simulink model "gm_sampleModel1448_3_sub"  (R2023a)
settings: Solver=VariableStepAuto  StartTime=0.0  StopTime=10.0  RelTol=1e-3
libraries: simulink x1
settings Model: Creator=user1  LastModifiedBy=user1
settings OptimizationCC: BlockReduction=off  ConditionallyExecuteInputs=off
settings DebuggingCC: InheritedTsInSrcMsg=none

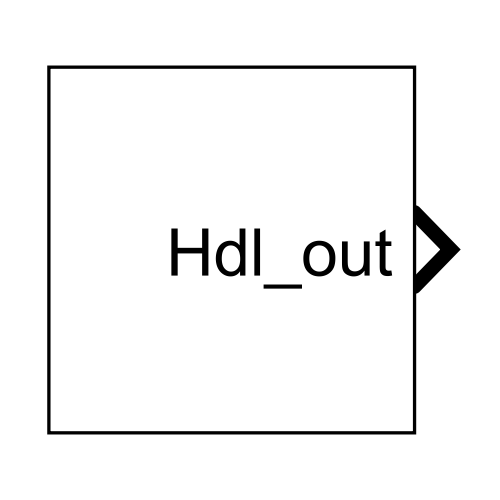
[thumbnail: Simulink's stored preview of the top-level diagram]
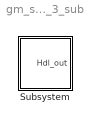
== system gm_sampleModel1448_3_sub ==
  Subsystem : Subsystem

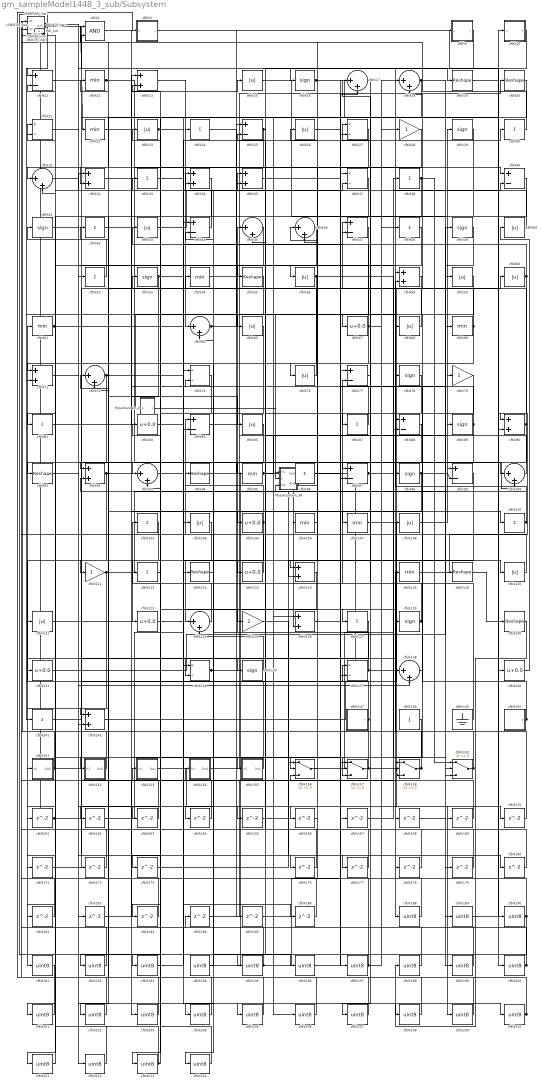
== system gm_sampleModel1448_3_sub/Subsystem ==
  Mysubsystem_3 : Subsystem
  Mysubsystem_38 : Subsystem
  cfblk10 : Subsystem  mask(Detect Rise Positive){vinit=double(0), InputProcessing=Elements as channels (sample based), OutDataTypeStr=uint8}
      mask prompts: vinit "Simulink:masks:InitialCondition_MP"; InputProcessing "Simulink:masks:InputProcessing_MP"; OutDataTypeStr "Simulink:masks:OutputDataType_MP"
      mask help: Simulink:masks:DetectRisePositive_MD
      mask init:
      | InputProcessing = 'Elements as channels (sample based)';
      | OutDataTypeStr = 'uint8';
      | vinit = double(0);
      mask TypeOptions InputProcessing: Simulink:masks:ColumnsAsChannelsFrameBased | Simulink:masks:ElementsAsChannelsSampleBased
      mask TypeOptions OutDataTypeStr: Simulink:masks:uint8 | Simulink:masks:boolean
      mask Display: fprintf('U > 0\n&  NOT\nU/z > 0')
  cfblk{17..18,31,45..46,64,72,93,100,124,138} (11 alike) : Sum  Inputs=|++  OutDataTypeStr=uint8
  cfblk101_inst : Subsystem
  cfblk102_inst : Subsystem
  cfblk{24,30,33,38,42,48,52,81,87,96,103,110,113,127,141} (15 alike) : Sum  Inputs=+  OutDataTypeStr=uint8
  cfblk{15,23,26,43,50,56,59..60,65,68,76,85,104,108,120..121} (16 alike) : Abs  OutDataTypeStr=uint8  SaturateOnIntegerOverflow=off
  cfblk{67,83,105,115,123,131,140} (7 alike) : Bias  Bias=0.0  SaturateOnIntegerOverflow=off
  cfblk{12,22,54,61,69,95,106..107,118} (9 alike) : MinMax  OutDataTypeStr=uint8
  cfblk{11,25,40,44,47,77,84,88,97,99} (10 alike) : Sum  Inputs=+-  OutDataTypeStr=uint8
  cfblk{28,79,112,125} (4 alike) : Gain  OutDataTypeStr=uint8
  cfblk{19..20,55,91,94,114,119,130} (8 alike) : Reshape
  cfblk{13,32,34..35,58,71,90,92,116,126,142} (11 alike) : Sum  OutDataTypeStr=uint8
  cfblk117_inst : Subsystem
  cfblk122_inst : Subsystem
  cfblk{16,29,41,49,53,78,89,98,128,135} (10 alike) : Signum
  cfblk129_inst : Subsystem
  cfblk{21,27,37,74,134,137} (6 alike) : Product  Inputs=*/  OutDataTypeStr=uint8  RndMeth=Zero  SaturateOnIntegerOverflow=on
  cfblk136_inst : Subsystem
  cfblk139_inst : Subsystem
  cfblk147 : Subsystem  mask(Counter Free-Running){NumBits=double(16), tsamp=double(-1)}
      mask prompts: NumBits "Simulink:masks:NumberOfBits_MP"; tsamp "Simulink:masks:SampleTime_MP"
      mask help: Simulink:masks:CounterFreeRunning_MD
  cfblk148 : Constant  OutDataTypeStr=uint8  SampleTime=-1
  cfblk149 : Ground
  cfblk14_inst : Subsystem
  cfblk150 : Subsystem  mask(Counter Free-Running){NumBits=double(16), tsamp=double(-1)}
      mask prompts: NumBits "Simulink:masks:NumberOfBits_MP"; tsamp "Simulink:masks:SampleTime_MP"
      mask help: Simulink:masks:CounterFreeRunning_MD
  cfblk151 : Subsystem
  cfblk152 : Subsystem
  cfblk153 : Subsystem
  cfblk154 : Subsystem
  cfblk155 : Subsystem
  cfblk{156..159} (4 alike) : Switch  OutDataTypeStr=uint8  SaturateOnIntegerOverflow=off  InputSameDT=off
  cfblk{161..173,176..186} (24 alike) : Delay  SampleTime=1
  cfblk{188..214} (27 alike) : DataTypeConversion  OutDataTypeStr=uint8  SaturateOnIntegerOverflow=off  RndMeth=Floor
  cfblk2 : Logic  AllPortsSameDT=off  OutDataTypeStr=boolean
  cfblk3 : Subsystem  mask(Compare To Zero){relop=<=, OutDataTypeStr=uint8, ZeroCross=on}
      mask prompts: relop "Simulink:masks:Operator_MP"; OutDataTypeStr "Simulink:masks:OutputDataType_MP"; ZeroCross "Simulink:masks:EnableZerocrossingDetection_MP"
      mask help: Simulink:masks:CompareToZero_MD
      mask init:
      | OutDataTypeStr = 'uint8';
      | ZeroCross = 'on';
      | blkName = 'sampleModel1448_3_sub/Subsystem/cfblk3';
      | relop = '<=';
      | setValue = 'fixdt(0, 8)';
      mask TypeOptions relop: == | ~= | < | <= | >= | >
      mask TypeOptions OutDataTypeStr: Simulink:masks:uint8 | Simulink:masks:boolean
      mask Callback ZeroCross: sl('zeroCrossEnable', gcbh);
      mask Display: disp([relop,' 0'])
  cfblk36_inst : Subsystem
  cfblk6 : Constant  Value=0  OutDataTypeStr=uint8  SampleTime=1
  cfblk63_inst : Subsystem
  cfblk66_inst : Subsystem
  cfblk70_inst : Subsystem
  cfblk75_inst : Subsystem
  cfblk8 : Constant  Value=0  OutDataTypeStr=uint8  SampleTime=1
  cfblk82_inst : Subsystem
  cfblk9 : Subsystem  mask(Compare To Constant){relop=<=, const=double(3), OutDataTypeStr=uint8, ZeroCross=on}
      mask prompts: relop "Simulink:masks:Operator_MP"; const "Simulink:masks:ConstantValue_MP"; OutDataTypeStr "Simulink:masks:OutputDataType_MP"; ZeroCross "Simulink:masks:EnableZerocrossingDetection_MP"
      mask help: Simulink:masks:CompareToConstant_MD
      mask init:
      | OutDataTypeStr = 'uint8';
      | ZeroCross = 'on';
      | blkName = 'sampleModel1448_3_sub/Subsystem/cfblk9';
      | const = double(3);
      | const_str = '3.0';
      | const_val = double(3);
      | relop = '<=';
      | setValue = 'fixdt(0, 8)';
      | str = '<= 3';
      mask TypeOptions relop: == | ~= | < | <= | >= | >
      mask TypeOptions OutDataTypeStr: Simulink:masks:uint8 | Simulink:masks:boolean
      mask Callback ZeroCross: sl('zeroCrossEnable', gcbh);
      mask Display: disp(str)
  Hdl_out : Outport  OutDataTypeStr=uint8  SampleTime=1
  wires:
  Mysubsystem_3/1(Out1) -> Mysubsystem_38/2(u)
  Mysubsystem_38/1(Out1) -> cfblk194/1, cfblk126/2, cfblk106/1
  Mysubsystem_38/2(Out2) -> cfblk66_inst/1(in1)
  cfblk10/1(Y) -> cfblk188/1
  cfblk100/1 -> cfblk45/2
  cfblk101_inst/1(out1) -> cfblk193/1
  cfblk102_inst/1(out1) -> cfblk168/1, cfblk22/1
  cfblk103/1 -> cfblk123/1
  cfblk104/1 -> cfblk191/1
  cfblk105/1 -> cfblk84/1, cfblk124/1
  cfblk106/1 -> cfblk46/1
  cfblk107/1 -> cfblk209/1
  cfblk108/1 -> cfblk29/1
  cfblk11/1 -> cfblk126/1
  cfblk110/1 -> cfblk58/2, Mysubsystem_38/3(In3)
  cfblk112/1 -> cfblk99/1, cfblk151/1(In1)
  cfblk113/1 -> cfblk213/1
  cfblk114/1 -> cfblk134/2
  cfblk115/1 -> cfblk94/1
  cfblk116/1 -> cfblk173/1
  cfblk117_inst/1(out1) -> cfblk69/1
  cfblk118/1 -> cfblk90/1
  cfblk119/1 -> cfblk130/1
  cfblk12/1 -> cfblk67/1, cfblk100/2
  cfblk120/1 -> cfblk129_inst/1(in1)
  cfblk121/1 -> cfblk156/2
  cfblk122_inst/1(out1) -> cfblk197/1
  cfblk123/1 -> cfblk127/1
  cfblk124/1 -> cfblk103/1
  cfblk125/1 -> cfblk177/1
  cfblk126/1 -> cfblk167/1
  cfblk127/1 -> cfblk201/1
  cfblk128/1 -> cfblk77/2, cfblk27/1
  cfblk129_inst/1(out1) -> cfblk114/1
  cfblk13/1 -> cfblk64/1
  cfblk130/1 -> cfblk198/1
  cfblk131/1 -> cfblk59/1
  cfblk134/1 -> cfblk20/1, cfblk54/1
  cfblk135/1 -> cfblk124/2
  cfblk136_inst/1(out1) -> cfblk203/1
  cfblk137/1 -> cfblk45/1, cfblk34/1
  cfblk138/1 -> cfblk96/1
  cfblk139_inst/1(out1) -> cfblk200/1
  cfblk14_inst/1(out1) -> cfblk19/1, cfblk11/1
  cfblk140/1 -> cfblk50/1
  cfblk141/1 -> cfblk60/1
  cfblk142/1 -> cfblk49/1
  cfblk147/1(y) -> cfblk44/2, cfblk211/1
  cfblk148/1 -> cfblk157/3
  cfblk149/1 -> cfblk53/1
  cfblk15/1 -> cfblk189/1
  cfblk150/1(y) -> cfblk92/2, cfblk78/1
  cfblk151/1(Out1) -> cfblk75_inst/2(in2), cfblk176/1
  cfblk152/1(Out1) -> cfblk75_inst/1(in1)
  cfblk153/1(Out1) -> cfblk166/1
  cfblk154/1(Out1) -> cfblk88/1
  cfblk155/1(Out1) -> cfblk61/1
  cfblk156/1 -> cfblk38/1
  cfblk157/1 -> cfblk158/3, cfblk155/1(In1)
  cfblk158/1 -> cfblk70_inst/1(in1), cfblk31/2
  cfblk159/1 -> cfblk2/1, cfblk118/1
  cfblk16/1 -> cfblk27/2, cfblk179/1
  cfblk161/1 -> cfblk156/1, Hdl_out/1
  cfblk162/1 -> cfblk37/2
  cfblk163/1 -> cfblk72/1
  cfblk164/1 -> cfblk63_inst/2(in2)
  cfblk165/1 -> cfblk77/1
  cfblk166/1 -> cfblk46/2
  cfblk167/1 -> cfblk40/2
  cfblk168/1 -> cfblk199/1
  cfblk169/1 -> cfblk13/2
  cfblk17/1 -> cfblk87/1
  cfblk170/1 -> cfblk34/2
  cfblk171/1 -> cfblk137/1
  cfblk172/1 -> cfblk117_inst/2(in2)
  cfblk173/1 -> cfblk158/2
  cfblk176/1 -> cfblk64/2
  cfblk177/1 -> cfblk25/2
  cfblk178/1 -> cfblk70_inst/2(in2)
  cfblk179/1 -> cfblk93/2
  cfblk18/1 -> cfblk97/1, cfblk32/2, cfblk100/1, cfblk183/1, cfblk24/1
  cfblk180/1 -> cfblk134/1
  cfblk181/1 -> cfblk129_inst/2(in2)
  cfblk182/1 -> cfblk156/3
  cfblk183/1 -> cfblk36_inst/2(in2)
  cfblk184/1 -> cfblk17/2
  cfblk185/1 -> cfblk157/1
  cfblk186/1 -> cfblk2/2
  cfblk188/1 -> cfblk26/1
  cfblk189/1 -> cfblk10/1(U)
  cfblk19/1 -> cfblk140/1
  cfblk190/1 -> cfblk83/1, cfblk214/1
  cfblk191/1 -> cfblk3/1(u)
  cfblk192/1 -> cfblk66_inst/2(in2)
  cfblk193/1 -> cfblk74/1
  cfblk194/1 -> cfblk74/2
  cfblk195/1 -> cfblk97/2, cfblk36_inst/1(in1)
  cfblk196/1 -> cfblk79/1
  cfblk197/1 -> cfblk82_inst/1(in1), cfblk18/1, cfblk37/1
  cfblk198/1 -> cfblk122_inst/1(in1)
  cfblk199/1 -> cfblk122_inst/2(in2)
  cfblk2/1 -> cfblk157/2
  cfblk20/1 -> cfblk95/1
  cfblk200/1 -> cfblk117_inst/1(in1), cfblk184/1, cfblk154/1(In1)
  cfblk201/1 -> cfblk139_inst/1(in1)
  cfblk202/1 -> cfblk139_inst/2(in2)
  cfblk203/1 -> cfblk14_inst/1(in1)
  cfblk204/1 -> cfblk136_inst/1(in1)
  cfblk205/1 -> cfblk136_inst/2(in2)
  cfblk206/1 -> cfblk14_inst/2(in2)
  cfblk207/1 -> cfblk42/1
  cfblk208/1 -> cfblk102_inst/2(in2)
  cfblk209/1 -> cfblk33/1
  cfblk21/1 -> cfblk210/1
  cfblk210/1 -> cfblk102_inst/1(in1), cfblk101_inst/2(in2)
  cfblk211/1 -> cfblk21/1
  cfblk212/1 -> cfblk21/2
  cfblk213/1 -> cfblk11/2, cfblk153/1(In1)
  cfblk214/1 -> cfblk113/1
  cfblk22/1 -> cfblk104/1
  cfblk23/1 -> cfblk55/1, cfblk40/1
  cfblk24/1 -> cfblk107/1
  cfblk25/1 -> cfblk84/2, cfblk125/1
  cfblk26/1 -> cfblk68/1
  cfblk27/1 -> cfblk76/1
  cfblk28/1 -> cfblk31/1
  cfblk29/1 -> cfblk65/1
  cfblk3/1(y) -> cfblk190/1
  cfblk30/1 -> cfblk63_inst/1(in1)
  cfblk31/1 -> cfblk180/1
  cfblk32/1 -> cfblk85/1
  cfblk33/1 -> cfblk208/1
  cfblk34/1 -> cfblk131/1
  cfblk35/1 -> cfblk128/1
  cfblk36_inst/1(out1) -> cfblk121/1
  cfblk37/1 -> cfblk137/2
  cfblk38/1 -> cfblk71/1, cfblk159/1
  cfblk40/1 -> cfblk72/2
  cfblk41/1 -> cfblk172/1
  cfblk42/1 -> cfblk206/1
  cfblk43/1 -> cfblk25/1
  cfblk44/1 -> cfblk32/1
  cfblk45/1 -> cfblk171/1
  cfblk46/1 -> cfblk81/1
  cfblk47/1 -> cfblk71/2
  cfblk48/1 -> cfblk116/1
  cfblk49/1 -> cfblk159/2
  cfblk50/1 -> cfblk101_inst/1(in1)
  cfblk52/1 -> cfblk41/1
  cfblk53/1 -> cfblk56/1, cfblk205/1, cfblk142/1
  cfblk54/1 -> cfblk185/1
  cfblk55/1 -> Mysubsystem_3/1(In1)
  cfblk56/1 -> cfblk202/1, cfblk159/3
  cfblk58/1 -> Mysubsystem_38/1(In1)
  cfblk59/1 -> cfblk158/1
  cfblk6/1 -> cfblk138/1, cfblk169/1
  cfblk60/1 -> cfblk90/2, cfblk43/1
  cfblk61/1 -> cfblk115/1, cfblk186/1
  cfblk63_inst/1(out1) -> cfblk196/1
  cfblk64/1 -> cfblk108/1, cfblk9/1(u)
  cfblk65/1 -> cfblk162/1
  cfblk66_inst/1(out1) -> cfblk52/1
  cfblk67/1 -> cfblk44/1, cfblk28/1, cfblk181/1
  cfblk68/1 -> cfblk23/1
  cfblk69/1 -> cfblk18/2, cfblk164/1, cfblk163/1
  cfblk70_inst/1(out1) -> cfblk138/2
  cfblk71/1 -> cfblk165/1
  cfblk72/1 -> cfblk142/2, cfblk30/1
  cfblk74/1 -> cfblk192/1
  cfblk75_inst/1(out1) -> cfblk82_inst/2(in2), cfblk141/1
  cfblk76/1 -> cfblk12/1
  cfblk77/1 -> cfblk17/1
  cfblk78/1 -> cfblk207/1
  cfblk79/1 -> cfblk195/1
  cfblk8/1 -> cfblk93/1
  cfblk81/1 -> cfblk15/1
  cfblk82_inst/1(out1) -> cfblk58/1, cfblk16/1, cfblk182/1
  cfblk83/1 -> cfblk47/1
  cfblk84/1 -> cfblk178/1
  cfblk85/1 -> cfblk91/1
  cfblk87/1 -> cfblk13/1
  cfblk88/1 -> cfblk92/1
  cfblk89/1 -> cfblk35/1, cfblk161/1
  cfblk9/1(y) -> cfblk135/1
  cfblk90/1 -> cfblk47/2, cfblk204/1
  cfblk91/1 -> cfblk212/1
  cfblk92/1 -> cfblk112/1, cfblk110/1
  cfblk93/1 -> cfblk120/1
  cfblk94/1 -> cfblk98/1
  cfblk95/1 -> cfblk89/1, cfblk35/2
  cfblk96/1 -> cfblk170/1
  cfblk97/1 -> cfblk88/2, cfblk48/1
  cfblk98/1 -> cfblk99/2, cfblk119/1, cfblk105/1, cfblk152/1(In1)
  cfblk99/1 -> cfblk116/2

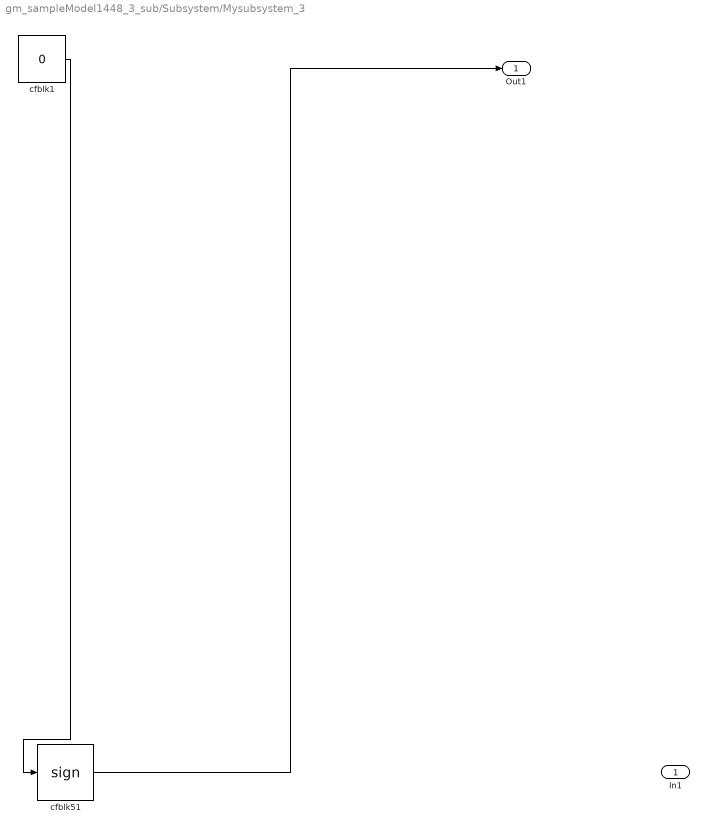
== system gm_sampleModel1448_3_sub/Subsystem/Mysubsystem_3 ==
  In1 : Inport  OutDataTypeStr=uint8  PortDimensions=1  SampleTime=1
  cfblk1 : Constant  Value=0  OutDataTypeStr=uint8  SampleTime=1
  cfblk51 : Signum
  Out1 : Outport  SampleTime=1
  wires:
  cfblk1/1 -> cfblk51/1
  cfblk51/1 -> Out1/1

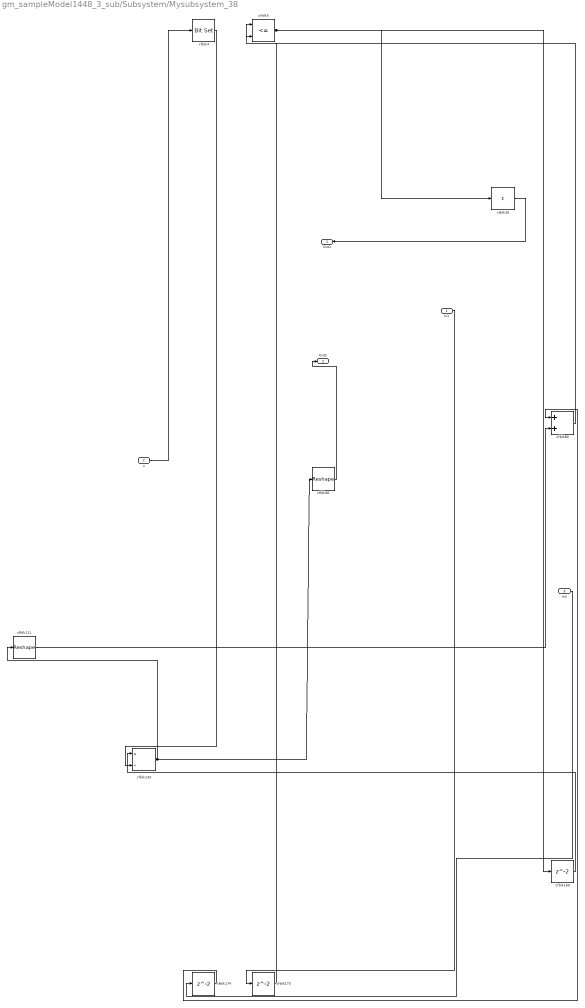
== system gm_sampleModel1448_3_sub/Subsystem/Mysubsystem_38 ==
  In1 : Inport  OutDataTypeStr=uint8  PortDimensions=1  SampleTime=1
  u : Inport  Port=2  OutDataTypeStr=uint8  PortDimensions=1  SampleTime=1
  In3 : Inport  Port=3  OutDataTypeStr=uint8  PortDimensions=1  SampleTime=1
  cfblk111 : Reshape
  cfblk133 : Product  Inputs=*/  RndMeth=Zero  SaturateOnIntegerOverflow=on
  cfblk160 : Delay  SampleTime=1
  cfblk174 : Delay  SampleTime=1
  cfblk175 : Delay  SampleTime=1
  cfblk39 : Sum  Inputs=+
  cfblk4 : simulink/Logic and Bit Operations/Bit Set  iBit=0
      settings: LibrarySourceBlock=|
      | hdlsllib/Logic and Bit
      | Operations/Bit Set
  cfblk5 : RelationalOperator  Operator=<=  OutDataTypeStr=boolean  InputSameDT=off
  cfblk80 : Sum
  cfblk86 : Reshape
  Out1 : Outport  SampleTime=1
  Out2 : Outport  Port=2  SampleTime=1
  wires:
  In1/1 -> cfblk175/1
  u/1 -> cfblk4/1
  In3/1 -> cfblk174/1
  cfblk111/1 -> cfblk80/2
  cfblk133/1 -> cfblk86/1, cfblk111/1
  cfblk160/1 -> cfblk133/1
  cfblk174/1 -> cfblk80/1
  cfblk175/1 -> cfblk5/1
  cfblk39/1 -> Out1/1
  cfblk4/1 -> cfblk133/2
  cfblk5/1 -> cfblk160/1, cfblk39/1
  cfblk80/1 -> cfblk5/2
  cfblk86/1 -> Out2/1

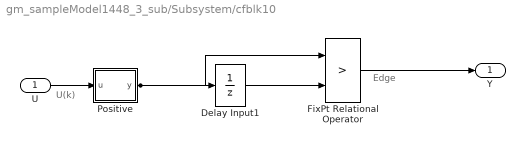
== system gm_sampleModel1448_3_sub/Subsystem/cfblk10 ==
  note: U(k)
  note: Edge
  U : Inport  OutDataTypeStr=uint8  SampleTime=1
  Delay Input1 : UnitDelay  Description=Store in Global RAM  DisableCoverage=on  InitialCondition=vinit  SampleTime=-1  HasFrameUpgradeWarning=on
  FixPt Relational Operator : RelationalOperator  Operator=>  OutDataTypeStr=fixdt(0, 8)  ZeroCross=off  InputSameDT=off
  Positive : Subsystem  mask(Compare To Zero){relop=>, OutDataTypeStr=boolean, ZeroCross=off}
      mask prompts: relop "Simulink:masks:Operator_MP"; OutDataTypeStr "Simulink:masks:OutputDataType_MP"; ZeroCross "Simulink:masks:EnableZerocrossingDetection_MP"
      mask help: Simulink:masks:CompareToZero_MD
      mask init:
      | OutDataTypeStr = 'boolean';
      | ZeroCross = 'off';
      | blkName = 'sampleModel1448_3_sub/Subsystem/cfblk10/Positive';
      | relop = '>';
      | setValue = 'boolean';
      mask TypeOptions relop: == | ~= | < | <= | >= | >
      mask TypeOptions OutDataTypeStr: Simulink:masks:uint8 | Simulink:masks:boolean
      mask Callback ZeroCross: sl('zeroCrossEnable', gcbh);
      mask Display: disp([relop,' 0'])
  Y : Outport  SampleTime=1
  wires:
  U/1 -> Positive/1(u)
  Delay Input1/1 -> FixPt Relational Operator/2
  FixPt Relational Operator/1 -> Y/1
  Positive/1(y) -> FixPt Relational Operator/1, Delay Input1/1

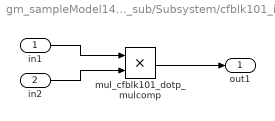
== system gm_sampleModel1448_3_sub/Subsystem/cfblk101_inst ==
  in1 : Inport  OutDataTypeStr=uint8  SampleTime=1
  in2 : Inport  Port=2  OutDataTypeStr=uint8  SampleTime=1
  mul_cfblk101_dotp_mulcomp : Product  Inputs=**  OutDataTypeStr=uint8  SampleTime=1
  out1 : Outport  OutDataTypeStr=uint8  SampleTime=1
  wires:
  in1/1 -> mul_cfblk101_dotp_mulcomp/1
  in2/1 -> mul_cfblk101_dotp_mulcomp/2
  mul_cfblk101_dotp_mulcomp/1 -> out1/1

== system gm_sampleModel1448_3_sub/Subsystem/cfblk102_inst ==
  in1 : Inport  OutDataTypeStr=uint8  SampleTime=1
  in2 : Inport  Port=2  OutDataTypeStr=uint8  SampleTime=1
  mul_cfblk102_dotp_mulcomp : Product  Inputs=**  OutDataTypeStr=uint8  SampleTime=1
  out1 : Outport  OutDataTypeStr=uint8  SampleTime=1
  wires:
  in1/1 -> mul_cfblk102_dotp_mulcomp/1
  in2/1 -> mul_cfblk102_dotp_mulcomp/2
  mul_cfblk102_dotp_mulcomp/1 -> out1/1

== system gm_sampleModel1448_3_sub/Subsystem/cfblk117_inst ==
  in1 : Inport  OutDataTypeStr=uint8  SampleTime=1
  in2 : Inport  Port=2  OutDataTypeStr=uint8  SampleTime=1
  mul_cfblk117_dotp_mulcomp : Product  Inputs=**  OutDataTypeStr=uint8  SampleTime=1
  out1 : Outport  OutDataTypeStr=uint8  SampleTime=1
  wires:
  in1/1 -> mul_cfblk117_dotp_mulcomp/1
  in2/1 -> mul_cfblk117_dotp_mulcomp/2
  mul_cfblk117_dotp_mulcomp/1 -> out1/1

== system gm_sampleModel1448_3_sub/Subsystem/cfblk122_inst ==
  in1 : Inport  OutDataTypeStr=uint8  SampleTime=1
  in2 : Inport  Port=2  OutDataTypeStr=uint8  SampleTime=1
  mul_cfblk122_dotp_mulcomp : Product  Inputs=**  OutDataTypeStr=uint8  SampleTime=1
  out1 : Outport  OutDataTypeStr=uint8  SampleTime=1
  wires:
  in1/1 -> mul_cfblk122_dotp_mulcomp/1
  in2/1 -> mul_cfblk122_dotp_mulcomp/2
  mul_cfblk122_dotp_mulcomp/1 -> out1/1

== system gm_sampleModel1448_3_sub/Subsystem/cfblk129_inst ==
  in1 : Inport  OutDataTypeStr=uint8  SampleTime=1
  in2 : Inport  Port=2  OutDataTypeStr=uint8  SampleTime=1
  mul_cfblk129_dotp_mulcomp : Product  Inputs=**  OutDataTypeStr=uint8  SampleTime=1
  out1 : Outport  OutDataTypeStr=uint8  SampleTime=1
  wires:
  in1/1 -> mul_cfblk129_dotp_mulcomp/1
  in2/1 -> mul_cfblk129_dotp_mulcomp/2
  mul_cfblk129_dotp_mulcomp/1 -> out1/1

== system gm_sampleModel1448_3_sub/Subsystem/cfblk136_inst ==
  in1 : Inport  OutDataTypeStr=uint8  SampleTime=1
  in2 : Inport  Port=2  OutDataTypeStr=uint8  SampleTime=1
  mul_cfblk136_dotp_mulcomp : Product  Inputs=**  OutDataTypeStr=uint8  SampleTime=1
  out1 : Outport  OutDataTypeStr=uint8  SampleTime=1
  wires:
  in1/1 -> mul_cfblk136_dotp_mulcomp/1
  in2/1 -> mul_cfblk136_dotp_mulcomp/2
  mul_cfblk136_dotp_mulcomp/1 -> out1/1

== system gm_sampleModel1448_3_sub/Subsystem/cfblk139_inst ==
  in1 : Inport  OutDataTypeStr=uint8  SampleTime=1
  in2 : Inport  Port=2  OutDataTypeStr=uint8  SampleTime=1
  mul_cfblk139_dotp_mulcomp : Product  Inputs=**  OutDataTypeStr=uint8  SampleTime=1
  out1 : Outport  OutDataTypeStr=uint8  SampleTime=1
  wires:
  in1/1 -> mul_cfblk139_dotp_mulcomp/1
  in2/1 -> mul_cfblk139_dotp_mulcomp/2
  mul_cfblk139_dotp_mulcomp/1 -> out1/1

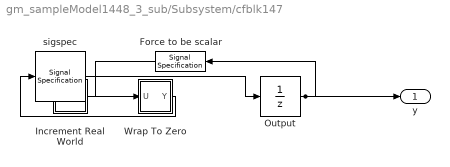
== system gm_sampleModel1448_3_sub/Subsystem/cfblk147 ==
  Force to be scalar : SignalSpecification  DisableCoverage=on  Dimensions=1
  Increment Real World : Subsystem  mask(Real World Value Increment){}
      mask help: Simulink:masks:RealWorldValueIncrement_MD
      mask Display: disp('V++')
  Output : UnitDelay  InitialCondition=0.0  SampleTime=tsamp  HasFrameUpgradeWarning=on
  Wrap To Zero : Subsystem  mask(Wrap To Zero){Threshold=double(65535)}
      mask prompts: Threshold "Simulink:masks:Threshold_MP"
      mask help: Simulink:masks:WrapToZero_MD
  sigspec : SignalSpecification  OutDataTypeStr=uint16  Dimensions=1
  y : Outport  SampleTime=1
  wires:
  Force to be scalar/1 -> Increment Real World/1(u)
  Increment Real World/1(y) -> Wrap To Zero/1(U)
  Output/1 -> Force to be scalar/1, y/1
  Wrap To Zero/1(Y) -> sigspec/1
  sigspec/1 -> Output/1

== system gm_sampleModel1448_3_sub/Subsystem/cfblk14_inst ==
  in1 : Inport  OutDataTypeStr=uint8  SampleTime=1
  in2 : Inport  Port=2  OutDataTypeStr=uint8  SampleTime=1
  mul_cfblk14_dotp_mulcomp : Product  Inputs=**  OutDataTypeStr=uint8  SampleTime=1
  out1 : Outport  OutDataTypeStr=uint8  SampleTime=1
  wires:
  in1/1 -> mul_cfblk14_dotp_mulcomp/1
  in2/1 -> mul_cfblk14_dotp_mulcomp/2
  mul_cfblk14_dotp_mulcomp/1 -> out1/1

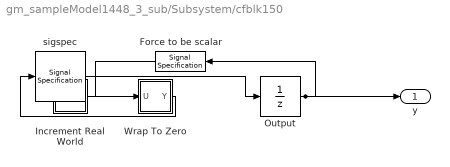
== system gm_sampleModel1448_3_sub/Subsystem/cfblk150 ==
  Force to be scalar : SignalSpecification  DisableCoverage=on  Dimensions=1
  Increment Real World : Subsystem  mask(Real World Value Increment){}
      mask help: Simulink:masks:RealWorldValueIncrement_MD
      mask Display: disp('V++')
  Output : UnitDelay  InitialCondition=0.0  SampleTime=tsamp  HasFrameUpgradeWarning=on
  Wrap To Zero : Subsystem  mask(Wrap To Zero){Threshold=double(65535)}
      mask prompts: Threshold "Simulink:masks:Threshold_MP"
      mask help: Simulink:masks:WrapToZero_MD
  sigspec : SignalSpecification  OutDataTypeStr=uint16  Dimensions=1
  y : Outport  SampleTime=1
  wires:
  Force to be scalar/1 -> Increment Real World/1(u)
  Increment Real World/1(y) -> Wrap To Zero/1(U)
  Output/1 -> Force to be scalar/1, y/1
  Wrap To Zero/1(Y) -> sigspec/1
  sigspec/1 -> Output/1

== system gm_sampleModel1448_3_sub/Subsystem/cfblk151 ==
  In1 : Inport  OutDataTypeStr=uint8  PortDimensions=1  SampleTime=1
  Out1 : Outport  SampleTime=1
  wires:
  In1/1 -> Out1/1

== system gm_sampleModel1448_3_sub/Subsystem/cfblk152 ==
  In1 : Inport  OutDataTypeStr=uint8  PortDimensions=1  SampleTime=1
  Out1 : Outport  SampleTime=1
  wires:
  In1/1 -> Out1/1

== system gm_sampleModel1448_3_sub/Subsystem/cfblk153 ==
  In1 : Inport  OutDataTypeStr=uint8  PortDimensions=1  SampleTime=1
  Out1 : Outport  SampleTime=1
  wires:
  In1/1 -> Out1/1

== system gm_sampleModel1448_3_sub/Subsystem/cfblk154 ==
  In1 : Inport  OutDataTypeStr=uint8  PortDimensions=1  SampleTime=1
  Out1 : Outport  SampleTime=1
  wires:
  In1/1 -> Out1/1

== system gm_sampleModel1448_3_sub/Subsystem/cfblk155 ==
  In1 : Inport  OutDataTypeStr=uint8  PortDimensions=1  SampleTime=1
  Out1 : Outport  SampleTime=1
  wires:
  In1/1 -> Out1/1

== system gm_sampleModel1448_3_sub/Subsystem/cfblk3 ==
  u : Inport  OutDataTypeStr=uint8  SampleTime=1
  Compare : RelationalOperator  Operator=<=  OutDataTypeStr=fixdt(0, 8)
  Constant : Constant  DisableCoverage=on  Value=0  OutDataTypeStr=Inherit: Inherit via back propagation  SampleTime=-1  PreserveConstantTs=on
  y : Outport  SampleTime=1
  wires:
  u/1 -> Compare/1
  Compare/1 -> y/1
  Constant/1 -> Compare/2

== system gm_sampleModel1448_3_sub/Subsystem/cfblk36_inst ==
  in1 : Inport  OutDataTypeStr=uint8  SampleTime=1
  in2 : Inport  Port=2  OutDataTypeStr=uint8  SampleTime=1
  mul_cfblk36_dotp_mulcomp : Product  Inputs=**  OutDataTypeStr=uint8  SampleTime=1
  out1 : Outport  OutDataTypeStr=uint8  SampleTime=1
  wires:
  in1/1 -> mul_cfblk36_dotp_mulcomp/1
  in2/1 -> mul_cfblk36_dotp_mulcomp/2
  mul_cfblk36_dotp_mulcomp/1 -> out1/1

== system gm_sampleModel1448_3_sub/Subsystem/cfblk63_inst ==
  in1 : Inport  OutDataTypeStr=uint8  SampleTime=1
  in2 : Inport  Port=2  OutDataTypeStr=uint8  SampleTime=1
  mul_cfblk63_dotp_mulcomp : Product  Inputs=**  OutDataTypeStr=uint8  SampleTime=1
  out1 : Outport  OutDataTypeStr=uint8  SampleTime=1
  wires:
  in1/1 -> mul_cfblk63_dotp_mulcomp/1
  in2/1 -> mul_cfblk63_dotp_mulcomp/2
  mul_cfblk63_dotp_mulcomp/1 -> out1/1

== system gm_sampleModel1448_3_sub/Subsystem/cfblk66_inst ==
  in1 : Inport  OutDataTypeStr=uint8  SampleTime=1
  in2 : Inport  Port=2  OutDataTypeStr=uint8  SampleTime=1
  mul_cfblk66_dotp_mulcomp : Product  Inputs=**  OutDataTypeStr=uint8  SampleTime=1
  out1 : Outport  OutDataTypeStr=uint8  SampleTime=1
  wires:
  in1/1 -> mul_cfblk66_dotp_mulcomp/1
  in2/1 -> mul_cfblk66_dotp_mulcomp/2
  mul_cfblk66_dotp_mulcomp/1 -> out1/1

== system gm_sampleModel1448_3_sub/Subsystem/cfblk70_inst ==
  in1 : Inport  OutDataTypeStr=uint8  SampleTime=1
  in2 : Inport  Port=2  OutDataTypeStr=uint8  SampleTime=1
  mul_cfblk70_dotp_mulcomp : Product  Inputs=**  OutDataTypeStr=uint8  SampleTime=1
  out1 : Outport  OutDataTypeStr=uint8  SampleTime=1
  wires:
  in1/1 -> mul_cfblk70_dotp_mulcomp/1
  in2/1 -> mul_cfblk70_dotp_mulcomp/2
  mul_cfblk70_dotp_mulcomp/1 -> out1/1

== system gm_sampleModel1448_3_sub/Subsystem/cfblk75_inst ==
  in1 : Inport  OutDataTypeStr=uint8  SampleTime=1
  in2 : Inport  Port=2  OutDataTypeStr=uint8  SampleTime=1
  mul_cfblk75_dotp_mulcomp : Product  Inputs=**  OutDataTypeStr=uint8  SampleTime=1
  out1 : Outport  OutDataTypeStr=uint8  SampleTime=1
  wires:
  in1/1 -> mul_cfblk75_dotp_mulcomp/1
  in2/1 -> mul_cfblk75_dotp_mulcomp/2
  mul_cfblk75_dotp_mulcomp/1 -> out1/1

== system gm_sampleModel1448_3_sub/Subsystem/cfblk82_inst ==
  in1 : Inport  OutDataTypeStr=uint8  SampleTime=1
  in2 : Inport  Port=2  OutDataTypeStr=uint8  SampleTime=1
  mul_cfblk82_dotp_mulcomp : Product  Inputs=**  OutDataTypeStr=uint8  SampleTime=1
  out1 : Outport  OutDataTypeStr=uint8  SampleTime=1
  wires:
  in1/1 -> mul_cfblk82_dotp_mulcomp/1
  in2/1 -> mul_cfblk82_dotp_mulcomp/2
  mul_cfblk82_dotp_mulcomp/1 -> out1/1

== system gm_sampleModel1448_3_sub/Subsystem/cfblk9 ==
  u : Inport  OutDataTypeStr=uint8  SampleTime=1
  Compare : RelationalOperator  Operator=<=  OutDataTypeStr=fixdt(0, 8)
  Constant : Constant  DisableCoverage=on  Value=const  OutDataTypeStr=Inherit: Inherit via back propagation  SampleTime=-1
  y : Outport  SampleTime=1
  wires:
  u/1 -> Compare/1
  Compare/1 -> y/1
  Constant/1 -> Compare/2

== system gm_sampleModel1448_3_sub/Subsystem/cfblk10/Positive ==
  u : Inport  OutDataTypeStr=uint8  SampleTime=1
  Compare : RelationalOperator  Operator=>  OutDataTypeStr=boolean  ZeroCross=off
  Constant : Constant  DisableCoverage=on  Value=0  OutDataTypeStr=Inherit: Inherit via back propagation  SampleTime=-1  PreserveConstantTs=on
  y : Outport  SampleTime=1
  wires:
  u/1 -> Compare/1
  Compare/1 -> y/1
  Constant/1 -> Compare/2

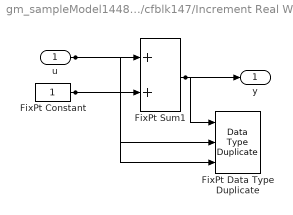
== system gm_sampleModel1448_3_sub/Subsystem/cfblk147/Increment Real World ==
  u : Inport  OutDataTypeStr=uint16  SampleTime=1
  FixPt Constant : Constant  DisableCoverage=on  OutDataTypeStr=Inherit: Inherit via back propagation  SampleTime=-1
  FixPt Data Type Duplicate : DataTypeDuplicate  DisableCoverage=on  NumInputPorts=3
  FixPt Sum1 : Sum  InputSameDT=on  OutDataTypeStr=Inherit: Inherit via back propagation  LockScale=on
  y : Outport  SampleTime=1
  wires:
  u/1 -> FixPt Sum1/1, FixPt Data Type Duplicate/2
  FixPt Constant/1 -> FixPt Sum1/2, FixPt Data Type Duplicate/3
  FixPt Sum1/1 -> FixPt Data Type Duplicate/1, y/1

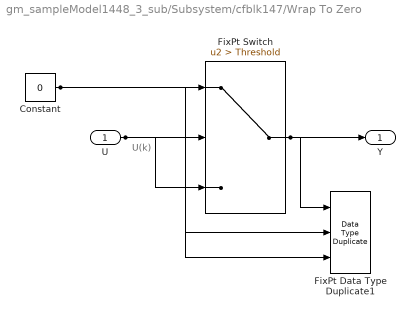
== system gm_sampleModel1448_3_sub/Subsystem/cfblk147/Wrap To Zero ==
  note: U(k)
  U : Inport  OutDataTypeStr=uint16  SampleTime=1
  Constant : Constant  DisableCoverage=on  Value=0  OutDataTypeStr=Inherit: Inherit via back propagation  SampleTime=-1
  FixPt Data Type Duplicate1 : DataTypeDuplicate  DisableCoverage=on  NumInputPorts=3
  FixPt Switch : Switch  Criteria=u2 > Threshold  Threshold=Threshold  OutDataTypeStr=Inherit: Inherit via back propagation  ZeroCross=off  SaturateOnIntegerOverflow=off  InputSameDT=off
  Y : Outport  SampleTime=1
  wires:
  U/1 -> FixPt Switch/3, FixPt Switch/2, FixPt Data Type Duplicate1/2
  Constant/1 -> FixPt Switch/1, FixPt Data Type Duplicate1/3
  FixPt Switch/1 -> FixPt Data Type Duplicate1/1, Y/1

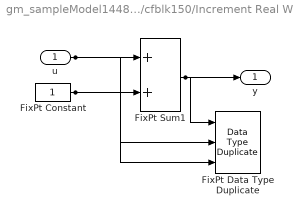
== system gm_sampleModel1448_3_sub/Subsystem/cfblk150/Increment Real World ==
  u : Inport  OutDataTypeStr=uint16  SampleTime=1
  FixPt Constant : Constant  DisableCoverage=on  OutDataTypeStr=Inherit: Inherit via back propagation  SampleTime=-1
  FixPt Data Type Duplicate : DataTypeDuplicate  DisableCoverage=on  NumInputPorts=3
  FixPt Sum1 : Sum  InputSameDT=on  OutDataTypeStr=Inherit: Inherit via back propagation  LockScale=on
  y : Outport  SampleTime=1
  wires:
  u/1 -> FixPt Sum1/1, FixPt Data Type Duplicate/2
  FixPt Constant/1 -> FixPt Sum1/2, FixPt Data Type Duplicate/3
  FixPt Sum1/1 -> FixPt Data Type Duplicate/1, y/1

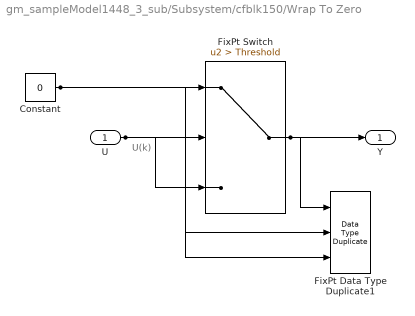
== system gm_sampleModel1448_3_sub/Subsystem/cfblk150/Wrap To Zero ==
  note: U(k)
  U : Inport  OutDataTypeStr=uint16  SampleTime=1
  Constant : Constant  DisableCoverage=on  Value=0  OutDataTypeStr=Inherit: Inherit via back propagation  SampleTime=-1
  FixPt Data Type Duplicate1 : DataTypeDuplicate  DisableCoverage=on  NumInputPorts=3
  FixPt Switch : Switch  Criteria=u2 > Threshold  Threshold=Threshold  OutDataTypeStr=Inherit: Inherit via back propagation  ZeroCross=off  SaturateOnIntegerOverflow=off  InputSameDT=off
  Y : Outport  SampleTime=1
  wires:
  U/1 -> FixPt Switch/3, FixPt Switch/2, FixPt Data Type Duplicate1/2
  Constant/1 -> FixPt Switch/1, FixPt Data Type Duplicate1/3
  FixPt Switch/1 -> FixPt Data Type Duplicate1/1, Y/1
